simulink model "WMMSupportingForcesGP2020a"  (R2020a)
settings: Solver=ode23t  StartTime=0.0  StopTime=inf  FixedStep=.001  RelTol=1e-3  AbsTol=1e-3
InitFcn:
  | InitializeSimulationGP
  | SimulationParametersGP
values from neighbouring files (symbols this model uses):
  B11_r_B11C = [0.23805608; 0.13201777; 0]    [InitializeSimulationGP.m]
  B11_r_B11Tc1 = [L11; 0; 0]    [InitializeSimulationGP.m]
  B11_Rot_Tc1 = eye(3)    [InitializeSimulationGP.m]
  B11cI = [0.28426000 -0.06487287 0;         -0.06487287  0.54237481 0;                   0  0          0.67891020]    [InitializeSimulationGP.m]
  B12_r_B12C = [0.60504569; 0.27199376; 0.00002484]    [InitializeSimulationGP.m]
  B12_r_B12Tc2 = [L12;0;0]    [InitializeSimulationGP.m]
  B12_Rot_Tc2 = eye(3)    [InitializeSimulationGP.m]
  B12cI = [1.18803886 -2.36786418 0.00280315;          -2.36786418 6.31493281 0.00022322;           0.00280315 0.00022322 7.40915161]    [InitializeSimulationGP.m]
  B31_r_B31C = [0.35781210 0 0]    [InitializeSimulationGP.m]
  B31_Rot_B41 = eye(3)    [InitializeSimulationGP.m]
  B31cI = diag([0.03150902 0.90735702 0.90763033])    [InitializeSimulationGP.m]
  B32_r_B32C = [0.35781210 0 0]    [InitializeSimulationGP.m]
  B32_Rot_B42 = eye(3)    [InitializeSimulationGP.m]
  B32cI = diag([0.03150902 0.90735702 0.90763033])    [InitializeSimulationGP.m]
  B41_r_B41C = [0.55785997 0 0]    [InitializeSimulationGP.m]
  B41_r_B41Tc1 = [lc1;0;0]    [InitializeSimulationGP.m]
  B41cI = diag([0.00370720 0.55759812 0.55785997])    [InitializeSimulationGP.m]
  B42_r_B42C = [0.55785997 0 0]    [InitializeSimulationGP.m]
  B42_r_B42Tc2 = [lc2; 0; 0]    [InitializeSimulationGP.m]
  B42cI = diag([0.00370720 0.55759812 0.55785997])    [InitializeSimulationGP.m]
  B52_r_B52C = [0 0 0.56802906]    [InitializeSimulationGP.m]
  B52_r_B52P32 = [lc3; 0; 0]    [InitializeSimulationGP.m]
  B52_Rot_P32 = eye(3)    [InitializeSimulationGP.m]
  B52cI = diag([0.91789884, 0.91790043, 0.00091463])    [InitializeSimulationGP.m]
  Bc1_r_Bc1B11 = [L1; 0; 0]    [InitializeSimulationGP.m]
  Bc1_r_Bc1B31 = [0;0;0]    [InitializeSimulationGP.m]
  Bc1_r_Bc1C = [0.14178771; 0.16555780; 0]    [InitializeSimulationGP.m]
  Bc1_V = [0;0;0;0;0;0]    [InitializeSimulationGP.m]
  Bc1cI = [+5.892211080 +5.476111360 -0.000019630;          +5.476111360 +28.66965601 -0.000024550;          -0.000019630 -0.000024550 +29.78955950]    [InitializeSimulationGP.m]
  Bc2_r_Bc2B12 = [L2;0;0]    [InitializeSimulationGP.m]
  Bc2_r_Bc2B32 = [0;0;0]    [InitializeSimulationGP.m]
  Bc2_r_Bc2C = [0.54319901; 0.10543875; 0]    [InitializeSimulationGP.m]
  Bc2cI = [0.48071390 0.52924041 0;          0.52924041 5.80912352 0;              0      0          5.97255351]    [InitializeSimulationGP.m]
  BC_r_BCBM = [xCA; yCA; zCA]    [SimulationParametersGP.m]
  BC_Rot_BM = eye(3)    [SimulationParametersGP.m]
  BCI = diag([100 1200 1000])    [SimulationParametersGP.m]
  beta1 = atan2d(374.261,935)*pi/180    [InitializeSimulationGP.m]
  beta2 = atan2d(45.757,373.313)*pi/180    [InitializeSimulationGP.m]
  beta3 = atan2d(139.50,1132.19)*pi/180    [InitializeSimulationGP.m]
  beta4 = atan2d(88.061,296.198)*pi/180    [InitializeSimulationGP.m]
  betaGround = 1e6    (= 1000000)    [SimulationParametersGP.m]
  BFL = 0.05    [SimulationParametersGP.m]
  BFR = 0.05    [SimulationParametersGP.m]
  BM_r_BMBMp = [0;0;0]    [SimulationParametersGP.m]
  BM_Rot_BMp = [cos(gamma) -sin(gamma) 0; sin(gamma) cos(gamma) 0; 0 0 1]    [SimulationParametersGP.m]
  BMp_r_BMpBc1 = [0.185;0;0.205]    [InitializeSimulationGP.m]
  BMp_Rot_Bc1 = [cos(alpha1) -sin(alpha1)  0;                  0            0       -1;                sin(alpha1)  cos(alpha1)  0]    [InitializeSimulationGP.m]
  BRL = 0.05    [SimulationParametersGP.m]
  BRR = 0.05    [SimulationParametersGP.m]
  cc = 0.0    (= 0)    [SimulationParametersGP.m]
  D22F = [0;0;0;0;0;0]    [InitializeSimulationGP.m]
  dT = 0.01    [SimulationParametersGP.m]
  g0 = 9.8066    [SimulationParametersGP.m]
  ground_stiffness = 1e8    (= 100000000)    [SimulationParametersGP.m]
  l1 = 1.15-cc    (= 1.15)    [SimulationParametersGP.m]
  L1 = 1.0071227324212    (= 1.00712273242)    [InitializeSimulationGP.m]
  L11 = 0.37610632101293    (= 0.376106321013)    [InitializeSimulationGP.m]
  L12 = 0.30901132665325    (= 0.309011326653)    [InitializeSimulationGP.m]
  l2 = 1.15+cc    (= 1.15)    [SimulationParametersGP.m]
  L2 = 1.132185817991    (= 1.13218581799)    [InitializeSimulationGP.m]
  lc1 = 0.745    [InitializeSimulationGP.m]
  lc2 = 0.745    [InitializeSimulationGP.m]
  mB11 = 25.52660174    [InitializeSimulationGP.m]
  mB12 = 33.92850233    [InitializeSimulationGP.m]
  mB31 = 17.36281648    [InitializeSimulationGP.m]
  mB32 = 17.36281648    [InitializeSimulationGP.m]
  mB41 = 10.34519231    [InitializeSimulationGP.m]
  mB42 = 10.34519231    [InitializeSimulationGP.m]
  mB52 = 6.73059863    [InitializeSimulationGP.m]
  mBC = 2200    [SimulationParametersGP.m]
  mBc1 = 307.29601379    [InitializeSimulationGP.m]
  mBc2 = 54.58702836    [InitializeSimulationGP.m]
  mFL = 60    [SimulationParametersGP.m]
  mFR = 60    [SimulationParametersGP.m]
  mP22 = 9.26136143    [InitializeSimulationGP.m]
  mP32 = 570.18877059    [InitializeSimulationGP.m]
  mRR = 60    [SimulationParametersGP.m]
  mw = mFL    (= 60)    [SimulationParametersGP.m]
  P22_r_P22C = [0.62192523 0 0]    [InitializeSimulationGP.m]
  P22_Rot_B52 = eye(3)    [InitializeSimulationGP.m]
  P22cI = diag([0.00662754, 1.48387017, 1.48398069])    [InitializeSimulationGP.m]
  P32_r_P32C = [0.25466704; -0.13034397; -0.01302248]    [InitializeSimulationGP.m]
  P32_r_P32D22 = [0.40499744871392; -0.13130517281345; -0.013385243295654]    [InitializeSimulationGP.m]
  P32_Rot_D22 = [1 0 0;              0 0.9707729441837 0.23999977258512;              0 -0.23999977258512 0.9707729441837]    [InitializeSimulationGP.m]
  P32cI = [46.81220713 0.38607676 -0.00453819;          0.38607676 71.92201786 -1.14320993;          -0.00453819 -1.14320993 67.38128576]    [InitializeSimulationGP.m]
  R0FL = 0.35    [SimulationParametersGP.m]
  R0FR = 0.35    [SimulationParametersGP.m]
  R0RL = 0.35    [SimulationParametersGP.m]
  R0RR = 0.35    [SimulationParametersGP.m]
  Rw = R0FL    (= 0.35)    [SimulationParametersGP.m]
  Tc1_r_Tc1Bc2 = [0.098495302558553; 0.01838181329939; 0]    [InitializeSimulationGP.m]
  Tc1_Rot_Bc2 = [cos(alpha2) -sin(alpha2) 0;                sin(alpha2)  cos(alpha2) 0;                0            0           1]    [InitializeSimulationGP.m]
  Tc2_r_Tc2P22 = [-0.048858374920227;0.36587359346146;0.035276938723102]    [InitializeSimulationGP.m]
  Tc2_Rot_P22 = [0.95853460763586 -0.27664713597974  0.0683942111482;                0.28497614981675  0.93051946315663 -0.23004808784757;                0                 0.23999977258511  0.9707729441837]    [InitializeSimulationGP.m]
  Th1A = 10*pi/180    (= 0.174532925199)    [InitializeSimulationGP.m]
  Th1B = 20*pi/180    (= 0.349065850399)    [InitializeSimulationGP.m]
  Th1f = 1    [InitializeSimulationGP.m]
  Th2A = 15*pi/180    (= 0.261799387799)    [InitializeSimulationGP.m]
  Th2B = -70*pi/180    (= -1.2217304764)    [InitializeSimulationGP.m]
  Th2f = 2    [InitializeSimulationGP.m]
  w = wFL    (= 0.875)    [SimulationParametersGP.m]
  W_r_WBc1 = [0.185;0;0.205]    [InitializeSimulationGP.m]
  W_Rot_Bc1 = [cos(alpha1) -sin(alpha1)  0;                  0            0       -1;                sin(alpha1)  cos(alpha1)  0]    [InitializeSimulationGP.m]
  x10 = 0.83    [InitializeSimulationGP.m]
  x20 = 0.83    [InitializeSimulationGP.m]
  x3A = 0.2    [InitializeSimulationGP.m]
  x3B = 0.3    [InitializeSimulationGP.m]
  x3f = 1    [InitializeSimulationGP.m]
  xCA = 0.5    [SimulationParametersGP.m]
  xf = [1;0;0;0;0;0]    [InitializeSimulationGP.m]
  yCA = 0    [SimulationParametersGP.m]
  zC = 0.45    [SimulationParametersGP.m]
  zCA = .25    (= 0.25)    [SimulationParametersGP.m]
  ztau = [0;0;0;0;0;1]    [InitializeSimulationGP.m]
undefined symbols (not defined in the file or in its folder): alphaFL_meas, alphaFR_meas, alphaRL_meas, alphaRR_meas, B11_V, B11Ftot, B12_U_Tc2, B12_V, B12Ftot, B31_r_B31B41, B31_V, B31FTot, B32_r_B32B42, B32_U_B42, B32_V, B32FTot, B41_V, B41FTot, B42_Rot_Tc2, B42_U_Tc2, B42_V, B42FTot, B52_U_P32, B52_V, B52Ftot, Bc1Tot, Bc2_Rot_B12, Bc2_Rot_B32, Bc2_U_B12, Bc2_U_B32, Bc2_V, Bc2Tot, betaC_meas, D22_V, deltaFL_cmd, deltaFL_meas, deltaFR_cmd, deltaFR_meas, deltaRL_cmd, deltaRL_meas, deltaRR_cmd, deltaRR_meas, dOmegaFL_meas, dOmegaFR_meas, dOmegaRL_meas, dOmegaRR_meas, dPsi_meas, dq1, dq11, dq12, dq2, dq21, dq22, dx1, dx2, Floor, FTot_S1, FTot_S2P, FTot_S2R, FzFL ... (+63)
libraries: sm_lib x94, nesl_utility x63, simulink x5
(part 10 of 11)

== system WMMSupportingForcesGP2020a/calc_wheel_velocities_and_sideslip_angles_from_meas/Hydraulic manipulator, calculation/AnalyticTotalForces/Structure 1/Subsystem9/Subsystem5 ==
  x : Inport
  Delay : Delay  InitialConditionSource=Input port  SampleTime=dT
      settings: InputPortMap=u0,p4
  Gain8 : Gain  Gain=1/(2*dT)
  Rate Transition : RateTransition  OutPortSampleTime=dT
  Sum4 : Sum  Inputs=|+-
  dx/dt : Outport
  wires:
  Gain8/1 -> dx/dt/1
  x/1 -> Rate Transition/1
  Delay/1 -> Sum4/2
  Sum4/1 -> Gain8/1
  Rate Transition/1 -> Sum4/1, Delay/1, Delay/2

== system WMMSupportingForcesGP2020a/calc_wheel_velocities_and_sideslip_angles_from_meas/Hydraulic manipulator, calculation/AnalyticTotalForces/Structure 1/Subsystem9/Subsystem6 ==
  x : Inport
  Delay : Delay  InitialConditionSource=Input port  SampleTime=dT
      settings: InputPortMap=u0,p4
  Gain8 : Gain  Gain=1/(2*dT)
  Rate Transition : RateTransition  OutPortSampleTime=dT
  Sum4 : Sum  Inputs=|+-
  dx/dt : Outport
  wires:
  Rate Transition/1 -> Delay/2, Delay/1, Sum4/1
  Sum4/1 -> Gain8/1
  Delay/1 -> Sum4/2
  x/1 -> Rate Transition/1
  Gain8/1 -> dx/dt/1

== system WMMSupportingForcesGP2020a/calc_wheel_velocities_and_sideslip_angles_from_meas/Hydraulic manipulator, calculation/AnalyticVelocities/Structure 1/GeomPropS1/LiftPistonStroke ==
  note: Pass to outputs...
  note: Process data...
  note: Derive piston stroke from q1-angle value...
  note: Get inputs...
  q1[rad] : Inport
  LiftPistonStroke : Fcn  Expr=sqrt(L1*L1+L11*L11+2*L1*L11*cos(u))-x10
  x1[m] : Outport
  wires:
  q1[rad]/1 -> [q1]
  [q1] -> LiftPistonStroke/1
  LiftPistonStroke/1 -> [x1]
  [x1] -> x1[m]/1

== system WMMSupportingForcesGP2020a/calc_wheel_velocities_and_sideslip_angles_from_meas/Hydraulic manipulator, calculation/AnalyticVelocities/Structure 1/GeomPropS1/Subsystem ==
  note: Pass to output...
  note: Process data...
  note: Get inputs...
  dq1 : Inport
  x1 : Inport  Port=2
  q1 : Inport  Port=3
  LiftPistonVelocity : MATLAB Function  TreatAsAtomicUnit=on
  dx1 : Outport
  wires:
  dq1/1 -> [dq1]
  [dq1] -> LiftPistonVelocity/1(dq1)
  x1/1 -> [x1]
  [x1] -> LiftPistonVelocity/2(x1)
  q1/1 -> [q1]
  [q1] -> LiftPistonVelocity/3(q1)
  LiftPistonVelocity/1(dx1) -> [dx1]  "dx1"
  [dx1] -> dx1/1

== system WMMSupportingForcesGP2020a/calc_wheel_velocities_and_sideslip_angles_from_meas/Hydraulic manipulator, calculation/AnalyticVelocities/Structure 1/GeomPropS1/Subsystem1 ==
  note: Pass to outputs...
  note: Process data...
  note: Get inputs...
  x1 : Inport
  q11 : Inport  Port=2
  dx1 : Inport  Port=3
  q11AngularVelocity : MATLAB Function  TreatAsAtomicUnit=on
  dq11 : Outport
  wires:
  x1/1 -> [x1]
  q11/1 -> [q11]
  dx1/1 -> [dx1]
  [x1] -> q11AngularVelocity/1(x1)  "x1"
  [q11] -> q11AngularVelocity/2(q11)  "q11"
  [dx1] -> q11AngularVelocity/3(dx1)  "dx1"
  q11AngularVelocity/1(dq11) -> [dq11]  "dq11"
  [dq11] -> dq11/1

== system WMMSupportingForcesGP2020a/calc_wheel_velocities_and_sideslip_angles_from_meas/Hydraulic manipulator, calculation/AnalyticVelocities/Structure 1/GeomPropS1/Subsystem2 ==
  note: Process data...
  note: Pass to outputs...
  note: Get inputs...
  x1 : Inport
  q12 : Inport  Port=2
  dx1 : Inport  Port=3
  q12AngularVelocity : MATLAB Function  TreatAsAtomicUnit=on
  dq12 : Outport
  wires:
  dx1/1 -> [dx1]
  q12/1 -> [q12]
  [dq12] -> dq12/1
  q12AngularVelocity/1(dq12) -> [dq12]  "dq12"
  x1/1 -> [x1]
  [q12] -> q12AngularVelocity/2(q12)  "q12"
  [x1] -> q12AngularVelocity/1(x1)  "x1"
  [dx1] -> q12AngularVelocity/3(dx1)  "dx1"

== system WMMSupportingForcesGP2020a/calc_wheel_velocities_and_sideslip_angles_from_meas/Hydraulic manipulator, calculation/AnalyticVelocities/Structure 1/GeomPropS1/q11-angle ==
  note: Pass to outputs...
  note: Process data...
  note: Get inputs...
  x1 : Inport
  Fcn : Fcn  Expr=-acos((L11*L11-(u+x10)*(u+x10)-L1*L1)/(-2*(u+x10)*L1))
  q11 : Outport
  wires:
  x1/1 -> [x1]
  [x1] -> Fcn/1
  Fcn/1 -> [q11]
  [q11] -> q11/1

== system WMMSupportingForcesGP2020a/calc_wheel_velocities_and_sideslip_angles_from_meas/Hydraulic manipulator, calculation/AnalyticVelocities/Structure 1/GeomPropS1/q12-angle ==
  note: Pass to outputs...
  note: Process data...
  note: Get inputs...
  x1 : Inport
  Fcn : Fcn  Expr=-acos((L1*L1-(u+x10)*(u+x10)-L11*L11)/(-2*(u+x10)*L11))
  q12 : Outport
  wires:
  x1/1 -> [x1]
  [x1] -> Fcn/1
  Fcn/1 -> [q12]
  [q12] -> q12/1

== system WMMSupportingForcesGP2020a/calc_wheel_velocities_and_sideslip_angles_from_meas/Hydraulic manipulator, calculation/AnalyticVelocities/Structure 1/GeomPropS1/q1Derivative ==
  note: Pass to outputs...
  note: Process data...
  note: Get inputs...
  q1 : Inport
  Subsystem2 : Subsystem
  dq1 : Outport
  wires:
  q1/1 -> [q1]  "q1"
  [q1] -> Subsystem2/1(x)  "q1"
  [dq1] -> dq1/1
  Subsystem2/1(dx/dt) -> [dq1]  "dq1"

== system WMMSupportingForcesGP2020a/calc_wheel_velocities_and_sideslip_angles_from_meas/Hydraulic manipulator, calculation/AnalyticVelocities/Structure 2 (Prismatic segment)/GeomPropS2P/Subsystem2 ==
  x : Inport
  Delay : Delay  InitialConditionSource=Input port  SampleTime=dT
      settings: InputPortMap=u0,p4
  Gain8 : Gain  Gain=1/(2*dT)
  Rate Transition : RateTransition  OutPortSampleTime=dT
  Sum4 : Sum  Inputs=|+-
  dx/dt : Outport
  wires:
  Rate Transition/1 -> Delay/2, Delay/1, Sum4/1
  Sum4/1 -> Gain8/1
  Delay/1 -> Sum4/2
  x/1 -> Rate Transition/1
  Gain8/1 -> dx/dt/1

== system WMMSupportingForcesGP2020a/calc_wheel_velocities_and_sideslip_angles_from_meas/Hydraulic manipulator, calculation/AnalyticVelocities/Structure 2 (Revolute segment)/GeomPropS2R/Subsystem4 ==
  note: Pass to outputs...
  note: Process data...
  note: Get inputs...
  x2 : Inport
  q21 : Inport  Port=2
  dx2 : Inport  Port=3
  q21AngularVelocity : MATLAB Function  TreatAsAtomicUnit=on
  dq21 : Outport
  wires:
  x2/1 -> [x2]  "x2"
  q21/1 -> [q21]  "q21"
  dx2/1 -> [dx2]  "dx2"
  [x2] -> q21AngularVelocity/1(x2)  "x2"
  q21AngularVelocity/1(dq21) -> [dq21]  "dq21"
  [dq21] -> dq21/1  "dq21"
  [dx2] -> q21AngularVelocity/2(dx2)  "dx2"
  [q21] -> q21AngularVelocity/3(q21)  "q21"

== system WMMSupportingForcesGP2020a/calc_wheel_velocities_and_sideslip_angles_from_meas/Hydraulic manipulator, calculation/AnalyticVelocities/Structure 2 (Revolute segment)/GeomPropS2R/Subsystem5 ==
  note: Process data...
  note: Pass to outputs...
  note: Get inputs...
  x2 : Inport
  q22 : Inport  Port=2
  dx2 : Inport  Port=3
  q22AngularVelocity : MATLAB Function  TreatAsAtomicUnit=on
  dq22 : Outport
  wires:
  dx2/1 -> [dx2]  "dx2"
  q22/1 -> [q22]  "q22"
  [dq22] -> dq22/1  "dq22"
  q22AngularVelocity/1(dq22) -> [dq22]  "dq22"
  x2/1 -> [x2]  "x2"
  [x2] -> q22AngularVelocity/1(x2)  "x2"
  [dx2] -> q22AngularVelocity/2(dx2)  "dx2"
  [q22] -> q22AngularVelocity/3(q22)  "q22"

== system WMMSupportingForcesGP2020a/calc_wheel_velocities_and_sideslip_angles_from_meas/Hydraulic manipulator, calculation/AnalyticVelocities/Structure 2 (Revolute segment)/GeomPropS2R/TiltPistonStroke ==
  note: Process data...
  note: Derive the tilt piston stroke from q2-angle value...
  note: Get inputs...
  note: Pass to outputs...
  q2[rad] : Inport
  TiltPistonStroke : Fcn  Expr=sqrt(L2*L2+L12*L12+2*L2*L12*cos(u))-x20
  x2[m] : Outport
  wires:
  [q2] -> TiltPistonStroke/1
  TiltPistonStroke/1 -> [x2]
  [x2] -> x2[m]/1
  q2[rad]/1 -> [q2]

== system WMMSupportingForcesGP2020a/calc_wheel_velocities_and_sideslip_angles_from_meas/Hydraulic manipulator, calculation/AnalyticVelocities/Structure 2 (Revolute segment)/GeomPropS2R/TiltPistonVelocity ==
  note: Pass to output...
  note: Process data...
  note: Get inputs...
  dq2 : Inport
  x2 : Inport  Port=2
  q2 : Inport  Port=3
  TiltPistonVelocity : MATLAB Function  TreatAsAtomicUnit=on
  dx2 : Outport
  wires:
  dq2/1 -> [dq2]  "dq2"
  [dq2] -> TiltPistonVelocity/3(dq2)  "dq2"
  x2/1 -> [x2]  "x2"
  [x2] -> TiltPistonVelocity/1(x2)  "x2"
  q2/1 -> [q2]  "q2"
  [q2] -> TiltPistonVelocity/2(q2)  "q2"
  [dx2] -> dx2/1  "dx2"
  TiltPistonVelocity/1(dx2) -> [dx2]  "dx2"

== system WMMSupportingForcesGP2020a/calc_wheel_velocities_and_sideslip_angles_from_meas/Hydraulic manipulator, calculation/AnalyticVelocities/Structure 2 (Revolute segment)/GeomPropS2R/q21-angle ==
  note: Pass to outputs...
  note: Process data...
  note: Get inputs...
  x2 : Inport
  Fcn : Fcn  Expr=-acos((L12*L12-(u+x20)*(u+x20)-L2*L2)/(-2*(u+x20)*L2))
  q21 : Outport
  wires:
  x2/1 -> [x2]
  [q21] -> q21/1
  [x2] -> Fcn/1
  Fcn/1 -> [q21]

== system WMMSupportingForcesGP2020a/calc_wheel_velocities_and_sideslip_angles_from_meas/Hydraulic manipulator, calculation/AnalyticVelocities/Structure 2 (Revolute segment)/GeomPropS2R/q22-angle ==
  note: Get inputs...
  note: Process data...
  note: Pass to outputs...
  x2 : Inport
  Fcn : Fcn  Expr=-acos((L2*L2-(u+x20)*(u+x20)-L12*L12)/(-2*(u+x20)*L12))
  q22 : Outport
  wires:
  [q22] -> q22/1
  Fcn/1 -> [q22]
  [x2] -> Fcn/1
  x2/1 -> [x2]

== system WMMSupportingForcesGP2020a/calc_wheel_velocities_and_sideslip_angles_from_meas/Hydraulic manipulator, calculation/AnalyticVelocities/Structure 2 (Revolute segment)/GeomPropS2R/q2Derivative ==
  note: Pass to outputs...
  note: Process data...
  note: Get inputs...
  q2 : Inport
  Subsystem2 : Subsystem
  dq2 : Outport
  wires:
  q2/1 -> [q2]  "q2"
  [q2] -> Subsystem2/1(x)  "q2"
  [dq2] -> dq2/1  "dq2"
  Subsystem2/1(dx/dt) -> [dq2]  "dq2"

== system WMMSupportingForcesGP2020a/calc_wheel_velocities_and_sideslip_angles_from_meas/Hydraulic manipulator, calculation/AnalyticVelocities/Structure 1/GeomPropS1/q1Derivative/Subsystem2 ==
  x : Inport
  Delay : Delay  InitialConditionSource=Input port  SampleTime=dT
      settings: InputPortMap=u0,p4
  Gain8 : Gain  Gain=1/(2*dT)
  Rate Transition : RateTransition  OutPortSampleTime=dT
  Sum4 : Sum  Inputs=|+-
  dx/dt : Outport
  wires:
  Rate Transition/1 -> Delay/2, Delay/1, Sum4/1
  Sum4/1 -> Gain8/1
  Delay/1 -> Sum4/2
  x/1 -> Rate Transition/1
  Gain8/1 -> dx/dt/1

== system WMMSupportingForcesGP2020a/calc_wheel_velocities_and_sideslip_angles_from_meas/Hydraulic manipulator, calculation/AnalyticVelocities/Structure 2 (Revolute segment)/GeomPropS2R/q2Derivative/Subsystem2 ==
  x : Inport
  Delay : Delay  InitialConditionSource=Input port  SampleTime=dT
      settings: InputPortMap=u0,p4
  Gain8 : Gain  Gain=1/(2*dT)
  Rate Transition : RateTransition  OutPortSampleTime=dT
  Sum4 : Sum  Inputs=|+-
  dx/dt : Outport
  wires:
  Rate Transition/1 -> Delay/2, Delay/1, Sum4/1
  Sum4/1 -> Gain8/1
  Delay/1 -> Sum4/2
  x/1 -> Rate Transition/1
  Gain8/1 -> dx/dt/1

== matlab function WMMSupportingForcesGP2020a/calc_wheel_velocities_and_sideslip_angles_from_meas/Hydraulic manipulator, calculation/AnalyticVelocities/Structure 1/GeomPropS1/Subsystem1/q11AngularVelocity ==
  data: x1 input; q11 input; dx1 input; dq11 output; L1 parameter; x10 parameter
function dq11 = dq11(x1, q11, dx1, L1, x10)

dq11 = -((x1+x10)-L1*cos(q11))/((x1+x10)*L1*sin(q11))*dx1;

== matlab function WMMSupportingForcesGP2020a/Mobile Manipulator in Simscape/WFL_kinematic_quantities/lateralForceFL ==
  data: FzFL input; alphaFL input; FyFL output
function FyFL = latForceFL(FzFL, alphaFL)

Dy = 0.5;
Ey = -0.9;
By = -11.37;
Cy = 1.33;

FyFL = Dy*FzFL*sin(Cy*atan(By*alphaFL - Ey*(By*alphaFL - atan(By*alphaFL))));

== matlab function WMMSupportingForcesGP2020a/calc_wheel_velocities_and_sideslip_angles_from_meas/Hydraulic manipulator, calculation/AnalyticVelocities/Structure 1/GeomPropS1/Subsystem2/q12AngularVelocity ==
  data: x1 input; q12 input; dx1 input; dq12 output; L11 parameter; x10 parameter
function dq12 = dq12(x1, q12, dx1, L11, x10)

dq12 = -((x1+x10)-L11*cos(q12))/((x1+x10)*L11*sin(q12))*dx1;

== matlab function WMMSupportingForcesGP2020a/Mobile Manipulator in Simscape/WFL_kinematic_quantities/longitudinalForceFL ==
  data: FzFL input; kappaFL input; FxFL output
function FxFL = longForceFL(FzFL, kappaFL)


% Fz0 = 4000;
% 
% dfz = (FzFL - Fz0)/FzFL;
% 
% pHx1 = 2.1585E-4;
% pHx2 = 0.0011538;
% SHx = (pHx1 + pHx2*dfz);
% kappax = kappaFL + SHx;
% 
% pDx1 = 1.0422;
% pDx2 = -0.0827;
% mux = pDx1 + pDx2*dfz;
% Dx = mux*FzFL;
% pCx1 = 1.579;
% Cx = pCx1;
% pEx1 = 0.11185;
% pEx2 = 0.3127;
% pEx3 = 0;
% pEx4 = 0.001603;
% Ex = (pEx1 + pEx2*dfz + pEx3*dfz^2)*(1 - pEx4*sign(kappax));
% pKx1 = 21.69;
% pKx2 = 13.774;
% pKx3 = -0.4119;
% Kxkappa = (pKx1 + pKx2*dfz)*exp(pKx3*dfz)*FzFL;
% Bx = Kxkappa/(Cx*Dx);
% pVx1 = 1.5973E-5;
% pVx2 = 1.043E-4;
% SVx = (pVx1 + pVx2*dfz)*FzFL;
% 
% FxFL = Dx*sin(Cx*atan(Bx*kappax - Ex*(Bx*kappax - atan(Bx*kappax)))) + 0*SVx;

Dx = 0.5;
Ex = 0;
Cx = 1.6;
Bx = 12.5;

FxFL = FzFL*Dx*sin(Cx*atan(Bx*kappaFL - Ex*(Bx*kappaFL - atan(Bx*kappaFL))));

== matlab function WMMSupportingForcesGP2020a/Mobile Manipulator in Simscape/WFR_kinematic_quantities/longitudinalForceFR ==
  data: FzFR input; kappaFR input; FxFR output
function FxFR = longForceFR(FzFR, kappaFR)


% Fz0 = 4000;
% 
% dfz = (FzFR - Fz0)/FzFR;
% 
% pHx1 = 2.1585E-4;
% pHx2 = 0.0011538;
% SHx = (pHx1 + pHx2*dfz);
% kappax = kappaFR + SHx;
% 
% pDx1 = 1.0422;
% pDx2 = -0.0827;
% mux = pDx1 + pDx2*dfz;
% Dx = mux*FzFR;
% pCx1 = 1.579;
% Cx = pCx1;
% pEx1 = 0.11185;
% pEx2 = 0.3127;
% pEx3 = 0;
% pEx4 = 0.001603;
% Ex = (pEx1 + pEx2*dfz + pEx3*dfz^2)*(1 - pEx4*sign(kappax));
% pKx1 = 21.69;
% pKx2 = 13.774;
% pKx3 = -0.4119;
% Kxkappa = (pKx1 + pKx2*dfz)*exp(pKx3*dfz)*FzFR;
% Bx = Kxkappa/(Cx*Dx);
% pVx1 = 1.5973E-5;
% pVx2 = 1.043E-4;
% SVx = (pVx1 + pVx2*dfz)*FzFR;
% 
% FxFR = Dx*sin(Cx*atan(Bx*kappax - Ex*(Bx*kappax - atan(Bx*kappax)))) + 0*SVx;

Dx = 0.5;
Ex = 0;
Cx = 1.6;
Bx = 12.5;

FxFR = FzFR*Dx*sin(Cx*atan(Bx*kappaFR - Ex*(Bx*kappaFR - atan(Bx*kappaFR))));

== matlab function WMMSupportingForcesGP2020a/Mobile Manipulator in Simscape/WRL_kinematic_quantities/lateralForceRL ==
  data: FzRL input; alphaRL input; FyRL output
function FyRL = latForceRL(FzRL, alphaRL)

Dy = 0.5;
Ey = -0.9;
By = -11.37;
Cy = 1.33;

FyRL = Dy*FzRL*sin(Cy*atan(By*alphaRL - Ey*(By*alphaRL - atan(By*alphaRL))));

== matlab function WMMSupportingForcesGP2020a/Mobile Manipulator in Simscape/WRL_kinematic_quantities/longitudinalForceRL ==
  data: FzRL input; kappaRL input; FxRL output
function FxRL = longForceRL(FzRL, kappaRL)

% 
% Fz0 = 4000;
% 
% dfz = (FzRL - Fz0)/FzRL;
% 
% pHx1 = 2.1585E-4;
% pHx2 = 0.0011538;
% SHx = (pHx1 + pHx2*dfz);
% kappax = kappaRL + SHx;
% 
% pDx1 = 1.0422;
% pDx2 = -0.0827;
% mux = pDx1 + pDx2*dfz;
% Dx = mux*FzRL;
% pCx1 = 1.579;
% Cx = pCx1;
% pEx1 = 0.11185;
% pEx2 = 0.3127;
% pEx3 = 0;
% pEx4 = 0.001603;
% Ex = (pEx1 + pEx2*dfz + pEx3*dfz^2)*(1 - pEx4*sign(kappax));
% pKx1 = 21.69;
% pKx2 = 13.774;
% pKx3 = -0.4119;
% Kxkappa = (pKx1 + pKx2*dfz)*exp(pKx3*dfz)*FzRL;
% Bx = Kxkappa/(Cx*Dx);
% pVx1 = 1.5973E-5;
% pVx2 = 1.043E-4;
% SVx = (pVx1 + pVx2*dfz)*FzRL;
% 
% FxRL = Dx*sin(Cx*atan(Bx*kappax - Ex*(Bx*kappax - atan(Bx*kappax)))) + 0*SVx;

Dx = 0.5;
Ex = 0;
Cx = 1.6;
Bx = 12.5;

FxRL = FzRL*Dx*sin(Cx*atan(Bx*kappaRL - Ex*(Bx*kappaRL - atan(Bx*kappaRL))));

== matlab function WMMSupportingForcesGP2020a/calc_wheel_velocities_and_sideslip_angles_from_meas/Hydraulic manipulator, calculation/AnalyticVelocities/Structure 1/PosVecsS1/B31_r_B31B41 ==
  data: x1 input; B31_r_B31B41 output; B31_r_B31B31p parameter
function B31_r_B31B41 = B31_r_B31B41(x1, B31_r_B31B31p)

% position vector of {B41} frame at lift piston tip w.r.t. {B31} frame at 
% lift cylinder connection point [m]
B31_r_B31B41 = B31_r_B31B31p + [x1;0;0];

== matlab function WMMSupportingForcesGP2020a/calc_wheel_velocities_and_sideslip_angles_from_meas/Hydraulic manipulator, calculation/AnalyticVelocities/Structure 1/RotMatsS1/B41_Rot_Tc1 ==
  data: q12 input; B41_Rot_Tc1 output
function B41_Rot_Tc1 = B41_Rot_Tc1(q12)

B41_Rot_Tc1 = [+cos(q12) -sin(q12) 0;...
               +sin(q12) +cos(q12) 0;...
                   0        0      1];

== matlab function WMMSupportingForcesGP2020a/calc_wheel_velocities_and_sideslip_angles_from_meas/Hydraulic manipulator, calculation/AnalyticVelocities/Structure 1/RotMatsS1/Bc1_Rot_B11 ==
  data: q1 input; Bc1_Rot_B11 output
function Bc1_Rot_B11 = Bc1_Rot_B11(q1)

Bc1_Rot_B11 = [+cos(q1) -sin(q1) 0;...
               +sin(q1) +cos(q1) 0;...
                  0        0     1];

== matlab function WMMSupportingForcesGP2020a/calc_wheel_velocities_and_sideslip_angles_from_meas/Hydraulic manipulator, calculation/AnalyticVelocities/Structure 1/RotMatsS1/Bc1_Rot_B31 ==
  data: q11 input; Bc1_Rot_B31 output
function Bc1_Rot_B31 = Bc1_Rot_B31(q11)

Bc1_Rot_B31 = [+cos(q11) -sin(q11) 0;...
               +sin(q11) +cos(q11) 0;...
                   0         0     1];

== matlab function WMMSupportingForcesGP2020a/calc_wheel_velocities_and_sideslip_angles_from_meas/Hydraulic manipulator, calculation/AnalyticVelocities/Structure 1/UMatsS1/B11_U_Tc1 ==
  data: B11_r_B11Tc1 input; B11_U_Tc1 output; B11_Rot_Tc1 input
function B11_U_Tc1 = B11_U_Tc1(B11_r_B11Tc1, B11_Rot_Tc1)

B11_U_Tc1 = [B11_Rot_Tc1,                    zeros(3);...
             dual(B11_r_B11Tc1)*B11_Rot_Tc1, B11_Rot_Tc1];
   
end
   
function dual_r = dual(ArAB)

dual_r = [0,  -ArAB(3), ArAB(2);...
          ArAB(3), 0, -ArAB(1);...
          -ArAB(2), ArAB(1), 0];

end

== matlab function WMMSupportingForcesGP2020a/calc_wheel_velocities_and_sideslip_angles_from_meas/Hydraulic manipulator, calculation/AnalyticVelocities/Structure 1/UMatsS1/B31_U_B41 ==
  data: B31_r_B31B41 input; B31_U_B41 output; B31_Rot_B41 input
function B31_U_B41 = B31_U_B41(B31_r_B31B41, B31_Rot_B41)

B31_U_B41 = [B31_Rot_B41,                    zeros(3);...
             dual(B31_r_B31B41)*B31_Rot_B41, B31_Rot_B41];
   
end
   
function dual_r = dual(ArAB)

dual_r = [0,  -ArAB(3), ArAB(2);...
          ArAB(3), 0, -ArAB(1);...
          -ArAB(2), ArAB(1), 0];

end

== matlab function WMMSupportingForcesGP2020a/calc_wheel_velocities_and_sideslip_angles_from_meas/Hydraulic manipulator, calculation/AnalyticVelocities/Structure 1/UMatsS1/B41_U_Tc1 ==
  data: B41_r_B41Tc1 input; B41_U_Tc1 output; B41_Rot_Tc1 input
function B41_U_Tc1 = B41_U_Tc1(B41_r_B41Tc1, B41_Rot_Tc1)

B41_U_Tc1 = [B41_Rot_Tc1,                    zeros(3);...
             dual(B41_r_B41Tc1)*B41_Rot_Tc1, B41_Rot_Tc1];
   
end
   
function dual_r = dual(ArAB)

dual_r = [0,  -ArAB(3), ArAB(2);...
          ArAB(3), 0, -ArAB(1);...
          -ArAB(2), ArAB(1), 0];

end

== matlab function WMMSupportingForcesGP2020a/calc_wheel_velocities_and_sideslip_angles_from_meas/Hydraulic manipulator, calculation/AnalyticTotalForces/Structure 1/MATLAB Function2 ==
  data: thetaB11 output; B11_r_B11C parameter; mB11 parameter; B11cI parameter
function thetaB11 = thetaB11(B11_r_B11C, mB11, B11cI)

rx = B11_r_B11C(1);
ry = B11_r_B11C(2);
rz = B11_r_B11C(3);

Ixx = B11cI(1,1);
Iyy = B11cI(2,2);
Izz = B11cI(3,3);
Iyz = B11cI(2,3);
Ixz = B11cI(1,3);
Ixy = B11cI(1,2);

t1 = rx*rx;
t2 = ry*ry;
t3 = rz*rz;
t4 = rx*mB11;

thetaB11 = [mB11; rx*mB11; ry*mB11; rz*mB11; t1*mB11; t2*mB11; t3*mB11; t4*ry - Ixy; t4*rz - Ixz; mB11*ry*rz - Iyz; Ixx; Iyy; Izz];

== matlab function WMMSupportingForcesGP2020a/calc_wheel_velocities_and_sideslip_angles_from_meas/Hydraulic manipulator, calculation/AnalyticTotalForces/Structure 1/MATLAB Function3 ==
  data: B11V input; B11a input; B11w input; B11dw input; B11_Rot_W input; Wg parameter; YB11 output
function YB11  = thetaBc1(B11V, B11a, B11w, B11dw, B11_Rot_W,  Wg)

vx = B11V(1);
vy = B11V(2);
vz = B11V(3);
ax = B11a(1);
ay = B11a(2);
az = B11a(3);
wx = B11w(1);
wy = B11w(2);
wz = B11w(3);
dwx = B11dw(1);
dwy = B11dw(2);
dwz = B11dw(3);
Bc1g = B11_Rot_W*Wg;
gx = Bc1g(1);
gy = Bc1g(2);
gz = Bc1g(3);

Y11 = ( ax + vz * wy - vy * wz  + gx);
t5 = (wy *  wy);
t6 = (wz * wz);
Y12 = -t5 - t6;
t7 = (wx * wy);
Y13 = (t7 - dwz);
t8 = (wx * wz);
Y14 = (t8 + dwy);
Y15 = 0;
Y16 = 0;
Y17 = 0;
Y18 = 0;
Y19 = 0;
Y110 = 0;
Y111 = 0;
Y112 = 0;
Y113 = 0;
Y21 = vx * wz - vz * wx + ay + gy;
Y22 = t7 + dwz;
t11 = wx * wx;
Y23 = -t11 - t6;
t12 = wy * wz;
Y24 = t12 - dwx;
Y25 = 0;
Y26 = 0;
Y27 = 0;
Y28 = 0;
Y29 = 0;
Y210 = 0;
Y211 = 0;
Y212 = 0;
Y213 = 0;
Y31 = -vx * wy + vy * wx + az + gz;
Y32 = t8 - dwy;
Y33 = t12 + dwx;
Y34 = -t11 - t5;
Y35 = 0;
Y36 = 0;
Y37 = 0;
Y38 = 0;
Y39 = 0;
Y310 = 0;
Y311 = 0;
Y312 = 0;
Y313 = 0;
Y41 = 0;
Y42 = 0;
Y43 = Y31;
Y44 = -Y21;
Y45 = 0;
Y46 = Y33;
Y47 = -Y24;
Y48 = Y32;
Y49 = -Y22;
Y410 = -t5 + t6;
Y411 = dwx;
Y412 = -t12;
Y413 = t12;
Y51 = 0;
Y52 = -Y31;
Y53 = 0;
Y54 = Y11;
Y55 = -Y32;
Y56 = 0;
Y57 = Y14;
Y58 = -Y33;
Y59 = t11 - t6;
Y510 = Y13;
Y511 = t8;
Y512 = dwy;
Y513 = -t8;
Y61 = 0;
Y62 = Y21;
Y63 = -Y11;
Y64 = 0;
Y65 = Y22;
Y66 = -Y13;
Y67 = 0;
Y68 = t5 - t11;
Y69 = Y24;
Y610 = -Y14;
Y611 = -t7;
Y612 = t7;
Y613 = dwz;

YB11 = [Y11 Y12 Y13 Y14 Y15 Y16 Y17 Y18 Y19 Y110 Y111 Y112 Y113;...
        Y21 Y22 Y23 Y24 Y25 Y26 Y27 Y28 Y29 Y210 Y211 Y212 Y213;...
        Y31 Y32 Y33 Y34 Y35 Y36 Y37 Y38 Y39 Y310 Y311 Y312 Y313;...
        Y41 Y42 Y43 Y44 Y45 Y46 Y47 Y48 Y49 Y410 Y411 Y412 Y413;...
        Y51 Y52 Y53 Y54 Y55 Y56 Y57 Y58 Y59 Y510 Y511 Y512 Y513;...
        Y61 Y62 Y63 Y64 Y65 Y66 Y67 Y68 Y69 Y610 Y611 Y612 Y613];

== matlab function WMMSupportingForcesGP2020a/calc_wheel_velocities_and_sideslip_angles_from_meas/Hydraulic manipulator, calculation/AnalyticTotalForces/Structure 1/MATLAB Function4 ==
  data: thetaB31 output; B31_r_B31C parameter; mB31 parameter; B31cI parameter
function thetaB31 = thetaB31(B31_r_B31C, mB31, B31cI)

rx = B31_r_B31C(1);
ry = B31_r_B31C(2);
rz = B31_r_B31C(3);

Ixx = B31cI(1,1);
Iyy = B31cI(2,2);
Izz = B31cI(3,3);
Iyz = B31cI(2,3);
Ixz = B31cI(1,3);
Ixy = B31cI(1,2);

t1 = rx*rx;
t2 = ry*ry;
t3 = rz*rz;
t4 = rx*mB31;

thetaB31 = [mB31; rx*mB31; ry*mB31; rz*mB31; t1*mB31; t2*mB31; t3*mB31; t4*ry - Ixy; t4*rz - Ixz; mB31*ry*rz - Iyz; Ixx; Iyy; Izz];

== matlab function WMMSupportingForcesGP2020a/calc_wheel_velocities_and_sideslip_angles_from_meas/Hydraulic manipulator, calculation/AnalyticVelocities/Structure 1/UMatsS1/Bc1_U_B11 ==
  data: Bc1_r_Bc1B11 input; Bc1_U_B11 output; Bc1_Rot_B11 input
function Bc1_U_B11 = Bc1_U_B11(Bc1_r_Bc1B11, Bc1_Rot_B11)

Bc1_U_B11 = [Bc1_Rot_B11,                    zeros(3);...
             dual(Bc1_r_Bc1B11)*Bc1_Rot_B11, Bc1_Rot_B11];
   
end
   
function dual_r = dual(ArAB)

dual_r = [0,  -ArAB(3), ArAB(2);...
          ArAB(3), 0, -ArAB(1);...
          -ArAB(2), ArAB(1), 0];

end

== matlab function WMMSupportingForcesGP2020a/calc_wheel_velocities_and_sideslip_angles_from_meas/Hydraulic manipulator, calculation/AnalyticTotalForces/Structure 1/MATLAB Function5 ==
  data: B31V input; B31a input; B31w input; B31dw input; B31_Rot_W input; Wg parameter; YB31 output
function YB31  = thetaBc1(B31V, B31a, B31w, B31dw, B31_Rot_W,  Wg)

vx = B31V(1);
vy = B31V(2);
vz = B31V(3);
ax = B31a(1);
ay = B31a(2);
az = B31a(3);
wx = B31w(1);
wy = B31w(2);
wz = B31w(3);
dwx = B31dw(1);
dwy = B31dw(2);
dwz = B31dw(3);
Bc1g = B31_Rot_W*Wg;
gx = Bc1g(1);
gy = Bc1g(2);
gz = Bc1g(3);

Y11 = ( ax + vz * wy - vy * wz  + gx);
t5 = (wy *  wy);
t6 = (wz * wz);
Y12 = -t5 - t6;
t7 = (wx * wy);
Y13 = (t7 - dwz);
t8 = (wx * wz);
Y14 = (t8 + dwy);
Y15 = 0;
Y16 = 0;
Y17 = 0;
Y18 = 0;
Y19 = 0;
Y110 = 0;
Y111 = 0;
Y112 = 0;
Y113 = 0;
Y21 = vx * wz - vz * wx + ay + gy;
Y22 = t7 + dwz;
t11 = wx * wx;
Y23 = -t11 - t6;
t12 = wy * wz;
Y24 = t12 - dwx;
Y25 = 0;
Y26 = 0;
Y27 = 0;
Y28 = 0;
Y29 = 0;
Y210 = 0;
Y211 = 0;
Y212 = 0;
Y213 = 0;
Y31 = -vx * wy + vy * wx + az + gz;
Y32 = t8 - dwy;
Y33 = t12 + dwx;
Y34 = -t11 - t5;
Y35 = 0;
Y36 = 0;
Y37 = 0;
Y38 = 0;
Y39 = 0;
Y310 = 0;
Y311 = 0;
Y312 = 0;
Y313 = 0;
Y41 = 0;
Y42 = 0;
Y43 = Y31;
Y44 = -Y21;
Y45 = 0;
Y46 = Y33;
Y47 = -Y24;
Y48 = Y32;
Y49 = -Y22;
Y410 = -t5 + t6;
Y411 = dwx;
Y412 = -t12;
Y413 = t12;
Y51 = 0;
Y52 = -Y31;
Y53 = 0;
Y54 = Y11;
Y55 = -Y32;
Y56 = 0;
Y57 = Y14;
Y58 = -Y33;
Y59 = t11 - t6;
Y510 = Y13;
Y511 = t8;
Y512 = dwy;
Y513 = -t8;
Y61 = 0;
Y62 = Y21;
Y63 = -Y11;
Y64 = 0;
Y65 = Y22;
Y66 = -Y13;
Y67 = 0;
Y68 = t5 - t11;
Y69 = Y24;
Y610 = -Y14;
Y611 = -t7;
Y612 = t7;
Y613 = dwz;

YB31 = [Y11 Y12 Y13 Y14 Y15 Y16 Y17 Y18 Y19 Y110 Y111 Y112 Y113;...
        Y21 Y22 Y23 Y24 Y25 Y26 Y27 Y28 Y29 Y210 Y211 Y212 Y213;...
        Y31 Y32 Y33 Y34 Y35 Y36 Y37 Y38 Y39 Y310 Y311 Y312 Y313;...
        Y41 Y42 Y43 Y44 Y45 Y46 Y47 Y48 Y49 Y410 Y411 Y412 Y413;...
        Y51 Y52 Y53 Y54 Y55 Y56 Y57 Y58 Y59 Y510 Y511 Y512 Y513;...
        Y61 Y62 Y63 Y64 Y65 Y66 Y67 Y68 Y69 Y610 Y611 Y612 Y613];

== matlab function WMMSupportingForcesGP2020a/calc_wheel_velocities_and_sideslip_angles_from_meas/Hydraulic manipulator, calculation/AnalyticTotalForces/Structure 2 (Prismatic segment)/MATLAB Function1 ==
  data: thetaB52 output; B52_r_B52C parameter; mB52 parameter; B52cI parameter
function thetaB52 = thetaB52(B52_r_B52C, mB52, B52cI)

rx = B52_r_B52C(1);
ry = B52_r_B52C(2);
rz = B52_r_B52C(3);

Ixx = B52cI(1,1);
Iyy = B52cI(2,2);
Izz = B52cI(3,3);
Iyz = B52cI(2,3);
Ixz = B52cI(1,3);
Ixy = B52cI(1,2);

t1 = rx*rx;
t2 = ry*ry;
t3 = rz*rz;
t4 = rx*mB52;

thetaB52 = [mB52; rx*mB52; ry*mB52; rz*mB52; t1*mB52; t2*mB52; t3*mB52; t4*ry - Ixy; t4*rz - Ixz; mB52*ry*rz - Iyz; Ixx; Iyy; Izz];

== matlab function WMMSupportingForcesGP2020a/calc_wheel_velocities_and_sideslip_angles_from_meas/Hydraulic manipulator, calculation/AnalyticTotalForces/Structure 1/MATLAB Function6 ==
  data: thetaB41 output; B41_r_B41C parameter; mB41 parameter; B41cI parameter
function thetaB41 = thetaB41(B41_r_B41C, mB41, B41cI)

rx = B41_r_B41C(1);
ry = B41_r_B41C(2);
rz = B41_r_B41C(3);

Ixx = B41cI(1,1);
Iyy = B41cI(2,2);
Izz = B41cI(3,3);
Iyz = B41cI(2,3);
Ixz = B41cI(1,3);
Ixy = B41cI(1,2);

t1 = rx*rx;
t2 = ry*ry;
t3 = rz*rz;
t4 = rx*mB41;

thetaB41 = [mB41; rx*mB41; ry*mB41; rz*mB41; t1*mB41; t2*mB41; t3*mB41; t4*ry - Ixy; t4*rz - Ixz; mB41*ry*rz - Iyz; Ixx; Iyy; Izz];

== matlab function WMMSupportingForcesGP2020a/calc_wheel_velocities_and_sideslip_angles_from_meas/Hydraulic manipulator, calculation/AnalyticTotalForces/Structure 1/MATLAB Function7 ==
  data: B41V input; B41a input; B41w input; B41dw input; B41_Rot_W input; Wg parameter; YB41 output
function YB41  = thetaB41(B41V, B41a, B41w, B41dw, B41_Rot_W,  Wg)

vx = B41V(1);
vy = B41V(2);
vz = B41V(3);
ax = B41a(1);
ay = B41a(2);
az = B41a(3);
wx = B41w(1);
wy = B41w(2);
wz = B41w(3);
dwx = B41dw(1);
dwy = B41dw(2);
dwz = B41dw(3);
Bc1g = B41_Rot_W*Wg;
gx = Bc1g(1);
gy = Bc1g(2);
gz = Bc1g(3);

Y11 = ( ax + vz * wy - vy * wz  + gx);
t5 = (wy *  wy);
t6 = (wz * wz);
Y12 = -t5 - t6;
t7 = (wx * wy);
Y13 = (t7 - dwz);
t8 = (wx * wz);
Y14 = (t8 + dwy);
Y15 = 0;
Y16 = 0;
Y17 = 0;
Y18 = 0;
Y19 = 0;
Y110 = 0;
Y111 = 0;
Y112 = 0;
Y113 = 0;
Y21 = vx * wz - vz * wx + ay + gy;
Y22 = t7 + dwz;
t11 = wx * wx;
Y23 = -t11 - t6;
t12 = wy * wz;
Y24 = t12 - dwx;
Y25 = 0;
Y26 = 0;
Y27 = 0;
Y28 = 0;
Y29 = 0;
Y210 = 0;
Y211 = 0;
Y212 = 0;
Y213 = 0;
Y31 = -vx * wy + vy * wx + az + gz;
Y32 = t8 - dwy;
Y33 = t12 + dwx;
Y34 = -t11 - t5;
Y35 = 0;
Y36 = 0;
Y37 = 0;
Y38 = 0;
Y39 = 0;
Y310 = 0;
Y311 = 0;
Y312 = 0;
Y313 = 0;
Y41 = 0;
Y42 = 0;
Y43 = Y31;
Y44 = -Y21;
Y45 = 0;
Y46 = Y33;
Y47 = -Y24;
Y48 = Y32;
Y49 = -Y22;
Y410 = -t5 + t6;
Y411 = dwx;
Y412 = -t12;
Y413 = t12;
Y51 = 0;
Y52 = -Y31;
Y53 = 0;
Y54 = Y11;
Y55 = -Y32;
Y56 = 0;
Y57 = Y14;
Y58 = -Y33;
Y59 = t11 - t6;
Y510 = Y13;
Y511 = t8;
Y512 = dwy;
Y513 = -t8;
Y61 = 0;
Y62 = Y21;
Y63 = -Y11;
Y64 = 0;
Y65 = Y22;
Y66 = -Y13;
Y67 = 0;
Y68 = t5 - t11;
Y69 = Y24;
Y610 = -Y14;
Y611 = -t7;
Y612 = t7;
Y613 = dwz;

YB41 = [Y11 Y12 Y13 Y14 Y15 Y16 Y17 Y18 Y19 Y110 Y111 Y112 Y113;...
        Y21 Y22 Y23 Y24 Y25 Y26 Y27 Y28 Y29 Y210 Y211 Y212 Y213;...
        Y31 Y32 Y33 Y34 Y35 Y36 Y37 Y38 Y39 Y310 Y311 Y312 Y313;...
        Y41 Y42 Y43 Y44 Y45 Y46 Y47 Y48 Y49 Y410 Y411 Y412 Y413;...
        Y51 Y52 Y53 Y54 Y55 Y56 Y57 Y58 Y59 Y510 Y511 Y512 Y513;...
        Y61 Y62 Y63 Y64 Y65 Y66 Y67 Y68 Y69 Y610 Y611 Y612 Y613];

== matlab function WMMSupportingForcesGP2020a/calc_wheel_velocities_and_sideslip_angles_from_meas/Hydraulic manipulator, calculation/AnalyticVelocities/Structure 1/UMatsS1/Bc1_U_B31 ==
  data: Bc1_r_Bc1B31 input; Bc1_U_B31 output; Bc1_Rot_B31 input
function Bc1_U_B31 = Bc1_U_B31(Bc1_r_Bc1B31, Bc1_Rot_B31)

Bc1_U_B31 = [Bc1_Rot_B31,                    zeros(3);...
             dual(Bc1_r_Bc1B31)*Bc1_Rot_B31, Bc1_Rot_B31];
   
end
   
function dual_r = dual(ArAB)

dual_r = [0,  -ArAB(3), ArAB(2);...
          ArAB(3), 0, -ArAB(1);...
          -ArAB(2), ArAB(1), 0];

end

== matlab function WMMSupportingForcesGP2020a/calc_wheel_velocities_and_sideslip_angles_from_meas/Hydraulic manipulator, calculation/AnalyticVelocities/Structure 1/UMatsS1/Tc1_U_Bc2 ==
  data: Tc1_r_Tc1Bc2 input; Tc1_U_Bc2 output; Tc1_Rot_Bc2 input
function Tc1_U_Bc2 = Tc1_U_Bc2(Tc1_r_Tc1Bc2, Tc1_Rot_Bc2)

Tc1_U_Bc2 = [Tc1_Rot_Bc2,                    zeros(3);...
             dual(Tc1_r_Tc1Bc2)*Tc1_Rot_Bc2, Tc1_Rot_Bc2];
   
end
   
function dual_r = dual(ArAB)

dual_r = [0,  -ArAB(3), ArAB(2);...
          ArAB(3), 0, -ArAB(1);...
          -ArAB(2), ArAB(1), 0];

end

== matlab function WMMSupportingForcesGP2020a/calc_wheel_velocities_and_sideslip_angles_from_meas/Hydraulic manipulator, calculation/AnalyticVelocities/Structure 2 (Prismatic segment)/PosVecsS2P/P22_r_P22B52 ==
  data: x3 input; P22_r_P22B52 output; P22_r_P22P22p parameter
function P22_r_P22B52 = P22_r_P22B52(x3, P22_r_P22P22p)

% position vector of {B41} frame at lift piston tip w.r.t. {B31} frame at 
% lift cylinder connection point [m]
P22_r_P22B52 = P22_r_P22P22p + [x3; 0; 0];

== matlab function WMMSupportingForcesGP2020a/calc_wheel_velocities_and_sideslip_angles_from_meas/Hydraulic manipulator, calculation/AnalyticVelocities/Structure 2 (Prismatic segment)/UMatsS2P/B52_U_P32 ==
  data: B52_r_B52B32 input; B52_U_P32 output; B52_Rot_B32 input
function B52_U_P32 = B52_U_P32(B52_r_B52B32, B52_Rot_B32)

B52_U_P32 = [B52_Rot_B32,                    zeros(3);...
             dual(B52_r_B52B32)*B52_Rot_B32, B52_Rot_B32];
   
end
   
function dual_r = dual(ArAB)

dual_r = [0,  -ArAB(3), ArAB(2);...
          ArAB(3), 0, -ArAB(1);...
          -ArAB(2), ArAB(1), 0];

end

== matlab function WMMSupportingForcesGP2020a/calc_wheel_velocities_and_sideslip_angles_from_meas/Hydraulic manipulator, calculation/AnalyticVelocities/Structure 2 (Prismatic segment)/UMatsS2P/P22_U_B52 ==
  data: P22_r_P22B52 input; P22_U_B52 output; P22_Rot_B52 input
function P22_U_B52 = P22_U_B52(P22_r_P22B52, P22_Rot_B52)

P22_U_B52 = [P22_Rot_B52,                    zeros(3);...
             dual(P22_r_P22B52)*P22_Rot_B52, P22_Rot_B52];
   
end
   
function dual_r = dual(ArAB)

dual_r = [0,  -ArAB(3), ArAB(2);...
          ArAB(3), 0, -ArAB(1);...
          -ArAB(2), ArAB(1), 0];

end

== matlab function WMMSupportingForcesGP2020a/calc_wheel_velocities_and_sideslip_angles_from_meas/Hydraulic manipulator, calculation/AnalyticVelocities/Structure 2 (Revolute segment)/PosVecsS2R/B32_r_B32B42 ==
  data: x2 input; B32_r_B32B42 output; B32_r_B32B32p parameter
function B32_r_B32B42 = B32_r_B32B42(x2, B32_r_B32B32p)

B32_r_B32B42 = B32_r_B32B32p + [x2;0;0];

== matlab function WMMSupportingForcesGP2020a/calc_wheel_velocities_and_sideslip_angles_from_meas/Hydraulic manipulator, calculation/AnalyticTotalForces/Structure 2 (Revolute segment)/MATLAB Function2 ==
  data: thetaB12 output; B12_r_B12C parameter; mB12 parameter; B12cI parameter
function thetaB12 = thetaB12(B12_r_B12C, mB12, B12cI)

rx = B12_r_B12C(1);
ry = B12_r_B12C(2);
rz = B12_r_B12C(3);

Ixx = B12cI(1,1);
Iyy = B12cI(2,2);
Izz = B12cI(3,3);
Iyz = B12cI(2,3);
Ixz = B12cI(1,3);
Ixy = B12cI(1,2);

t1 = rx*rx;
t2 = ry*ry;
t3 = rz*rz;
t4 = rx*mB12;

thetaB12 = [mB12; rx*mB12; ry*mB12; rz*mB12; t1*mB12; t2*mB12; t3*mB12; t4*ry - Ixy; t4*rz - Ixz; mB12*ry*rz - Iyz; Ixx; Iyy; Izz];

== matlab function WMMSupportingForcesGP2020a/calc_wheel_velocities_and_sideslip_angles_from_meas/Hydraulic manipulator, calculation/AnalyticTotalForces/Structure 2 (Revolute segment)/MATLAB Function4 ==
  data: thetaB32 output; B32_r_B32C parameter; mB32 parameter; B32cI parameter
function thetaB32 = thetaB32(B32_r_B32C, mB32, B32cI)

rx = B32_r_B32C(1);
ry = B32_r_B32C(2);
rz = B32_r_B32C(3);

Ixx = B32cI(1,1);
Iyy = B32cI(2,2);
Izz = B32cI(3,3);
Iyz = B32cI(2,3);
Ixz = B32cI(1,3);
Ixy = B32cI(1,2);

t1 = rx*rx;
t2 = ry*ry;
t3 = rz*rz;
t4 = rx*mB32;

thetaB32 = [mB32; rx*mB32; ry*mB32; rz*mB32; t1*mB32; t2*mB32; t3*mB32; t4*ry - Ixy; t4*rz - Ixz; mB32*ry*rz - Iyz; Ixx; Iyy; Izz];

== matlab function WMMSupportingForcesGP2020a/calc_wheel_velocities_and_sideslip_angles_from_meas/Hydraulic manipulator, calculation/AnalyticTotalForces/Structure 2 (Prismatic segment)/MATLAB Function6 ==
  data: thetaP22 output; P22_r_P22C parameter; mP22 parameter; P22cI parameter
function thetaP22 = thetaP22(P22_r_P22C, mP22, P22cI)

rx = P22_r_P22C(1);
ry = P22_r_P22C(2);
rz = P22_r_P22C(3);

Ixx = P22cI(1,1);
Iyy = P22cI(2,2);
Izz = P22cI(3,3);
Iyz = P22cI(2,3);
Ixz = P22cI(1,3);
Ixy = P22cI(1,2);

t1 = rx*rx;
t2 = ry*ry;
t3 = rz*rz;
t4 = rx*mP22;

thetaP22 = [mP22; rx*mP22; ry*mP22; rz*mP22; t1*mP22; t2*mP22; t3*mP22; t4*ry - Ixy; t4*rz - Ixz; mP22*ry*rz - Iyz; Ixx; Iyy; Izz];

== matlab function WMMSupportingForcesGP2020a/calc_wheel_velocities_and_sideslip_angles_from_meas/Hydraulic manipulator, calculation/AnalyticTotalForces/Structure 2 (Revolute segment)/MATLAB Function6 ==
  data: thetaB42 output; B42_r_B42C parameter; mB42 parameter; B42cI parameter
function thetaB42 = thetaB42(B42_r_B42C, mB42, B42cI)

rx = B42_r_B42C(1);
ry = B42_r_B42C(2);
rz = B42_r_B42C(3);

Ixx = B42cI(1,1);
Iyy = B42cI(2,2);
Izz = B42cI(3,3);
Iyz = B42cI(2,3);
Ixz = B42cI(1,3);
Ixy = B42cI(1,2);

t1 = rx*rx;
t2 = ry*ry;
t3 = rz*rz;
t4 = rx*mB42;

thetaB42 = [mB42; rx*mB42; ry*mB42; rz*mB42; t1*mB42; t2*mB42; t3*mB42; t4*ry - Ixy; t4*rz - Ixz; mB42*ry*rz - Iyz; Ixx; Iyy; Izz];

== matlab function WMMSupportingForcesGP2020a/calc_wheel_velocities_and_sideslip_angles_from_meas/Hydraulic manipulator, calculation/AnalyticTotalForces/Structure 2 (Revolute segment)/MATLAB Function ==
  data: thetaBc2 output; Bc2_r_Bc2C parameter; mBc2 parameter; Bc2cI parameter
function thetaBc2 = thetaBc2(Bc2_r_Bc2C, mBc2, Bc2cI)

rx = Bc2_r_Bc2C(1);
ry = Bc2_r_Bc2C(2);
rz = Bc2_r_Bc2C(3);

Ixx = Bc2cI(1,1);
Iyy = Bc2cI(2,2);
Izz = Bc2cI(3,3);
Iyz = Bc2cI(2,3);
Ixz = Bc2cI(1,3);
Ixy = Bc2cI(1,2);

t1 = rx*rx;
t2 = ry*ry;
t3 = rz*rz;
t4 = rx*mBc2;

thetaBc2 = [mBc2; rx*mBc2; ry*mBc2; rz*mBc2; t1*mBc2; t2*mBc2; t3*mBc2; t4*ry - Ixy; t4*rz - Ixz; mBc2*ry*rz - Iyz; Ixx; Iyy; Izz];

== matlab function WMMSupportingForcesGP2020a/calc_wheel_velocities_and_sideslip_angles_from_meas/Hydraulic manipulator, calculation/AnalyticTotalForces/Structure 2 (Revolute segment)/MATLAB Function3 ==
  data: B12V input; B12a input; B12w input; B12dw input; B12_Rot_W input; Wg parameter; YB12 output
function YB12  = thetaB12(B12V, B12a, B12w, B12dw, B12_Rot_W,  Wg)

vx = B12V(1);
vy = B12V(2);
vz = B12V(3);
ax = B12a(1);
ay = B12a(2);
az = B12a(3);
wx = B12w(1);
wy = B12w(2);
wz = B12w(3);
dwx = B12dw(1);
dwy = B12dw(2);
dwz = B12dw(3);
B12g = B12_Rot_W*Wg;
gx = B12g(1);
gy = B12g(2);
gz = B12g(3);

Y11 = ( ax + vz * wy - vy * wz  + gx);
t5 = (wy *  wy);
t6 = (wz * wz);
Y12 = -t5 - t6;
t7 = (wx * wy);
Y13 = (t7 - dwz);
t8 = (wx * wz);
Y14 = (t8 + dwy);
Y15 = 0;
Y16 = 0;
Y17 = 0;
Y18 = 0;
Y19 = 0;
Y110 = 0;
Y111 = 0;
Y112 = 0;
Y113 = 0;
Y21 = vx * wz - vz * wx + ay + gy;
Y22 = t7 + dwz;
t11 = wx * wx;
Y23 = -t11 - t6;
t12 = wy * wz;
Y24 = t12 - dwx;
Y25 = 0;
Y26 = 0;
Y27 = 0;
Y28 = 0;
Y29 = 0;
Y210 = 0;
Y211 = 0;
Y212 = 0;
Y213 = 0;
Y31 = -vx * wy + vy * wx + az + gz;
Y32 = t8 - dwy;
Y33 = t12 + dwx;
Y34 = -t11 - t5;
Y35 = 0;
Y36 = 0;
Y37 = 0;
Y38 = 0;
Y39 = 0;
Y310 = 0;
Y311 = 0;
Y312 = 0;
Y313 = 0;
Y41 = 0;
Y42 = 0;
Y43 = Y31;
Y44 = -Y21;
Y45 = 0;
Y46 = Y33;
Y47 = -Y24;
Y48 = Y32;
Y49 = -Y22;
Y410 = -t5 + t6;
Y411 = dwx;
Y412 = -t12;
Y413 = t12;
Y51 = 0;
Y52 = -Y31;
Y53 = 0;
Y54 = Y11;
Y55 = -Y32;
Y56 = 0;
Y57 = Y14;
Y58 = -Y33;
Y59 = t11 - t6;
Y510 = Y13;
Y511 = t8;
Y512 = dwy;
Y513 = -t8;
Y61 = 0;
Y62 = Y21;
Y63 = -Y11;
Y64 = 0;
Y65 = Y22;
Y66 = -Y13;
Y67 = 0;
Y68 = t5 - t11;
Y69 = Y24;
Y610 = -Y14;
Y611 = -t7;
Y612 = t7;
Y613 = dwz;

YB12 = [Y11 Y12 Y13 Y14 Y15 Y16 Y17 Y18 Y19 Y110 Y111 Y112 Y113;...
        Y21 Y22 Y23 Y24 Y25 Y26 Y27 Y28 Y29 Y210 Y211 Y212 Y213;...
        Y31 Y32 Y33 Y34 Y35 Y36 Y37 Y38 Y39 Y310 Y311 Y312 Y313;...
        Y41 Y42 Y43 Y44 Y45 Y46 Y47 Y48 Y49 Y410 Y411 Y412 Y413;...
        Y51 Y52 Y53 Y54 Y55 Y56 Y57 Y58 Y59 Y510 Y511 Y512 Y513;...
        Y61 Y62 Y63 Y64 Y65 Y66 Y67 Y68 Y69 Y610 Y611 Y612 Y613];

== matlab function WMMSupportingForcesGP2020a/calc_wheel_velocities_and_sideslip_angles_from_meas/Hydraulic manipulator, calculation/AnalyticTotalForces/Structure 2 (Revolute segment)/MATLAB Function5 ==
  data: B32V input; B32a input; B32w input; B32dw input; B32_Rot_W input; Wg parameter; YB32 output
function YB32  = thetaB32(B32V, B32a, B32w, B32dw, B32_Rot_W,  Wg)

vx = B32V(1);
vy = B32V(2);
vz = B32V(3);
ax = B32a(1);
ay = B32a(2);
az = B32a(3);
wx = B32w(1);
wy = B32w(2);
wz = B32w(3);
dwx = B32dw(1);
dwy = B32dw(2);
dwz = B32dw(3);
B32g = B32_Rot_W*Wg;
gx = B32g(1);
gy = B32g(2);
gz = B32g(3);

Y11 = ( ax + vz * wy - vy * wz  + gx);
t5 = (wy *  wy);
t6 = (wz * wz);
Y12 = -t5 - t6;
t7 = (wx * wy);
Y13 = (t7 - dwz);
t8 = (wx * wz);
Y14 = (t8 + dwy);
Y15 = 0;
Y16 = 0;
Y17 = 0;
Y18 = 0;
Y19 = 0;
Y110 = 0;
Y111 = 0;
Y112 = 0;
Y113 = 0;
Y21 = vx * wz - vz * wx + ay + gy;
Y22 = t7 + dwz;
t11 = wx * wx;
Y23 = -t11 - t6;
t12 = wy * wz;
Y24 = t12 - dwx;
Y25 = 0;
Y26 = 0;
Y27 = 0;
Y28 = 0;
Y29 = 0;
Y210 = 0;
Y211 = 0;
Y212 = 0;
Y213 = 0;
Y31 = -vx * wy + vy * wx + az + gz;
Y32 = t8 - dwy;
Y33 = t12 + dwx;
Y34 = -t11 - t5;
Y35 = 0;
Y36 = 0;
Y37 = 0;
Y38 = 0;
Y39 = 0;
Y310 = 0;
Y311 = 0;
Y312 = 0;
Y313 = 0;
Y41 = 0;
Y42 = 0;
Y43 = Y31;
Y44 = -Y21;
Y45 = 0;
Y46 = Y33;
Y47 = -Y24;
Y48 = Y32;
Y49 = -Y22;
Y410 = -t5 + t6;
Y411 = dwx;
Y412 = -t12;
Y413 = t12;
Y51 = 0;
Y52 = -Y31;
Y53 = 0;
Y54 = Y11;
Y55 = -Y32;
Y56 = 0;
Y57 = Y14;
Y58 = -Y33;
Y59 = t11 - t6;
Y510 = Y13;
Y511 = t8;
Y512 = dwy;
Y513 = -t8;
Y61 = 0;
Y62 = Y21;
Y63 = -Y11;
Y64 = 0;
Y65 = Y22;
Y66 = -Y13;
Y67 = 0;
Y68 = t5 - t11;
Y69 = Y24;
Y610 = -Y14;
Y611 = -t7;
Y612 = t7;
Y613 = dwz;

YB32 = [Y11 Y12 Y13 Y14 Y15 Y16 Y17 Y18 Y19 Y110 Y111 Y112 Y113;...
        Y21 Y22 Y23 Y24 Y25 Y26 Y27 Y28 Y29 Y210 Y211 Y212 Y213;...
        Y31 Y32 Y33 Y34 Y35 Y36 Y37 Y38 Y39 Y310 Y311 Y312 Y313;...
        Y41 Y42 Y43 Y44 Y45 Y46 Y47 Y48 Y49 Y410 Y411 Y412 Y413;...
        Y51 Y52 Y53 Y54 Y55 Y56 Y57 Y58 Y59 Y510 Y511 Y512 Y513;...
        Y61 Y62 Y63 Y64 Y65 Y66 Y67 Y68 Y69 Y610 Y611 Y612 Y613];

== matlab function WMMSupportingForcesGP2020a/Mobile Manipulator in Simscape/WRR_kinematic_quantities/lateralForceRR ==
  data: FzRR input; alphaRR input; FyRR output
function FyRR  = latForceRR(FzRR, alphaRR)

Dy = 0.5;
Ey = -0.9;
By = -11.37;
Cy = 1.33;

FyRR = Dy*FzRR*sin(Cy*atan(By*alphaRR - Ey*(By*alphaRR - atan(By*alphaRR))));

== matlab function WMMSupportingForcesGP2020a/Mobile Manipulator in Simscape/WRR_kinematic_quantities/longitudinalForceRR ==
  data: FzRR input; kappaRR input; FxRR output
function FxRR = longForceRR(FzRR, kappaRR)


% Fz0 = 4000;
% 
% dfz = (FzRR - Fz0)/FzRR;
% 
% pHx1 = 2.1585E-4;
% pHx2 = 0.0011538;
% SHx = (pHx1 + pHx2*dfz);
% kappax = kappaRR + SHx;
% 
% pDx1 = 1.0422;
% pDx2 = -0.0827;
% mux = pDx1 + pDx2*dfz;
% Dx = mux*FzRR;
% pCx1 = 1.579;
% Cx = pCx1;
% pEx1 = 0.11185;
% pEx2 = 0.3127;
% pEx3 = 0;
% pEx4 = 0.001603;
% Ex = (pEx1 + pEx2*dfz + pEx3*dfz^2)*(1 - pEx4*sign(kappax));
% pKx1 = 21.69;
% pKx2 = 13.774;
% pKx3 = -0.4119;
% Kxkappa = (pKx1 + pKx2*dfz)*exp(pKx3*dfz)*FzRR;
% Bx = Kxkappa/(Cx*Dx);
% pVx1 = 1.5973E-5;
% pVx2 = 1.043E-4;
% SVx = (pVx1 + pVx2*dfz)*FzRR;
% 
% FxRR = Dx*sin(Cx*atan(Bx*kappax - Ex*(Bx*kappax - atan(Bx*kappax)))) + 0*SVx;

Dx = 0.5;
Ex = 0;
Cx = 1.6;
Bx = 12.5;

FxRR =  FzRR*Dx*sin(Cx*atan(Bx*kappaRR - Ex*(Bx*kappaRR - atan(Bx*kappaRR))));

== matlab function WMMSupportingForcesGP2020a/Mobile Manipulator in Simscape/get_measurements/MATLAB Function ==
  data: u input; Theta output; Phi output; Psi output
function [Theta, Phi, Psi] = fcn(u)

Theta = atan(u(1,3)/u(3,3));
Phi = asin(-u(2,3));
Psi = atan(u(2,1)/u(2,2));
